simulink model "ANCfb"  (R2023b)
settings: Solver=ode3  StartTime=0.0  StopTime=10  RelTol=1e-3  EnableMultiTasking=on
libraries: matrix_library x52, dspadpt3 x31, raspberrypiAVlib x3
(part 1 of 2)
settings Model: FPTRunName=Active  ExtModeTrigDuration=2  Creator=aaron  LastModifiedBy=aaron
settings SolverCC: AlgebraicLoopSolver=TrustRegion  PositivePriorityOrder=on
settings DataIOCC: LimitDataPoints=on  SaveFormat=Array
settings OptimizationCC: ExpressionDepthLimit=2147483647  LifeSpan=Inf  MaxStackSize=64
settings DebuggingCC: UnderspecifiedInitializationDetection=Classic  MergeDetectMultiDrivingBlocksExec=none  FcnCallInpInsideContextMsg=warning  UnconnectedInputMsg=warning  UnconnectedOutputMsg=warning  UnconnectedLineMsg=warning  AllowSymbolicDim=off  StateNameClashWarn=warning  SubsystemReferenceDiagnosticForUnitTest=warning  SFUnexpectedBacktrackingDiag=warning  SFNoUnconditionalDefaultTransitionDiag=warning  SFExecutionAtInitializationDiag=none  ArithmeticOperatorsInVariantConditions=warning
settings HardwareCC: ProdBitPerPointer=32  ProdBitPerSizeT=32  ProdBitPerPtrDiffT=32  ProdLargestAtomicInteger=Long  ProdLargestAtomicFloat=Double  ProdWordSize=32  ProdHWDeviceType=ARM Compatible->ARM Cortex  UseEmbeddedCoderFeatures=off  UseSimulinkCoderFeatures=off
settings ModelReferenceCC: EnableRefExpFcnMdlSchedulingChecks=on  PropagateSignalLabelsOutOfModel=off
settings SFSimCC: SimUseLocalCustomCode=off  CustomCodeUndefinedFunction=UseInterfaceOnly
settings RTWCC: Description=Embedded Coder  SystemTargetFile=ert.tlc  HardwareBoard=Raspberry Pi  TemplateMakefile=ert_default_tmf  GenerateReport=on  RTWVerbose=off  RTWUseLocalCustomCode=off  Toolchain=GNU GCC Embedded Linux  BuildConfiguration=Faster Runs  LaunchReport=on
settings CodeAppCC: ForceParamTrailComments=on  OperatorAnnotations=on  StateflowObjectComments=on  MATLABSourceComments=on
settings ERTTargetCC: MultiwordLength=2048  ERTCustomFileBanners=off  SupportContinuousTime=on  SupportNonInlinedSFcns=on  RemoveResetFunc=off  SupportVariableSizeSignals=on  ModelStepFunctionPrototypeControlCompliant=off
settings ConfigComp: CovMetricSettings=dw  CovSaveCumulativeToWorkspaceVar=on  CovSaveSingleToWorkspaceVar=on  CovExternalEMLEnable=off  CovSFcnEnable=off

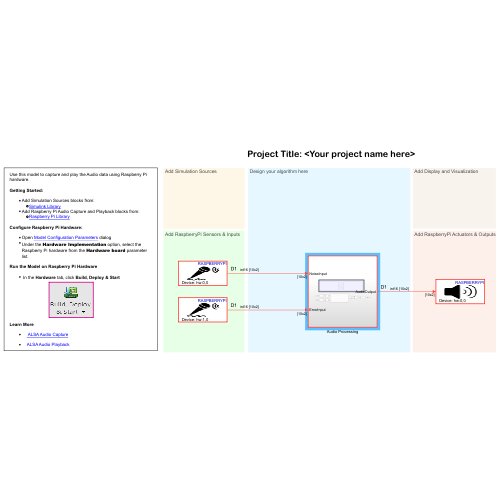
[thumbnail: Simulink's stored preview of the top-level diagram]
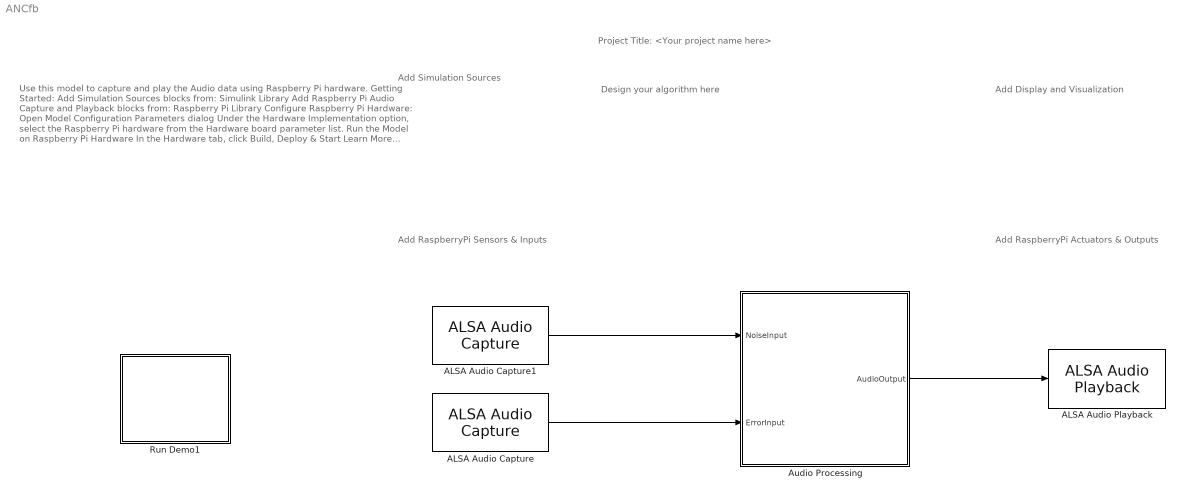
== system ANCfb ==
  note: Use this model to capture and play the Audio data using Raspberry Pi hardware.
      |
      | Getting Started:
      |
      | Add Simulation Sources blocks from:
      | Simulink Library
      | Add Raspberry Pi Audio Capture and Playback blocks from:
      | Raspberry Pi Library
      |
      | Configure Raspberry Pi Hardware:
      |
      | Open Model Configuration Parameters dialog
      | Under the Hardware Implementation option, select the Raspberry Pi hardware from the Hardware board parameter list.
      |
      | Run the Model on Raspberry Pi Hardware
      |
      | In the Hardware tab, click Build, Deploy & Start
      |
      | Learn More
      | ALSA Audio Capture
      | ALSA Audio Playback
  note: Add Simulation Sources
  note: Add Display and Visualization
  note: Design your algorithm here
  note: Add RaspberryPi Actuators & Outputs
  note: Project Title: <Your project name here>
  note: Add RaspberryPi Sensors & Inputs
  ALSA Audio Capture : raspberrypiAVlib/ALSA Audio Capture  deviceStr='hw:1,0'  DataBitDepth=16-bit integer  numberOfChannels=2  sampleRateEnum=44100  frameSize=10  QueueDuration=0.5  blockPlatform=Raspberry Pi
  ALSA Audio Capture1 : raspberrypiAVlib/ALSA Audio Capture  deviceStr='hw:0,0'  DataBitDepth=16-bit integer  numberOfChannels=2  sampleRateEnum=44100  frameSize=10  QueueDuration=0.5  blockPlatform=Raspberry Pi
  ALSA Audio Playback : raspberrypiAVlib/ALSA Audio Playback  deviceStr='hw:0,0'  sampleRateEnum=44100  queueDuration=0.5  blockPlatform=Raspberry Pi
  Audio Processing : Subsystem
  Run Demo1 : Subsystem  Description=Controls host-side RTDX processing.
      mask Display: pic=imread('raspberrypiBuildDeployAndStart.png');image(pic);
  wires:
  Audio Processing/1(AudioOutput) -> ALSA Audio Playback/1
  ALSA Audio Capture1/1 -> Audio Processing/1(NoiseInput)
  ALSA Audio Capture/1 -> Audio Processing/2(ErrorInput)

== system ANCfb/Audio Processing ==
  note: Unused Blocks
  NoiseInput : Inport
  ErrorInput : Inport  Port=2
  Data Type Conversion : DataTypeConversion  OutDataTypeStr=double  SaturateOnIntegerOverflow=off  RndMeth=Floor
  Data Type Conversion1 : DataTypeConversion  OutDataTypeStr=int16  SaturateOnIntegerOverflow=off  RndMeth=Floor  LockScale=on
  Data Type Conversion2 : DataTypeConversion  OutDataTypeStr=double  SaturateOnIntegerOverflow=off  RndMeth=Floor
  Frame Breakdown : Subsystem  TreatAsAtomicUnit=on
  Matrix Concatenate : Concatenate  Mode=Multidimensional array  ConcatenateDimension=2
  NoError : Subsystem  Commented=on  TreatAsAtomicUnit=on
  "Right Channel, exec" : Subsystem  Commented=on  TreatAsAtomicUnit=on
  Submatrix : matrix_library/Submatrix  RowSpan=All rows  RowStartMode=First  RowStartIndex=1  RowEndMode=Last  RowEndIndex=1  ColSpan=One column  ColStartMode=First  ColStartIndex=1  ColEndMode=Last  ColEndIndex=1
  Submatrix2 : matrix_library/Submatrix  RowSpan=All rows  RowStartMode=First  RowStartIndex=1  RowEndMode=Last  RowEndIndex=1  ColSpan=One column  ColStartMode=First  ColStartIndex=1  ColEndMode=Last  ColEndIndex=1
  AudioOutput : Outport
  wires:
  Data Type Conversion/1 -> Submatrix/1
  Submatrix/1 -> Frame Breakdown/1(Noise input (ref. mic.))
  NoiseInput/1 -> Data Type Conversion/1
  Data Type Conversion1/1 -> AudioOutput/1
  Frame Breakdown/1(Anti-noise output) -> Matrix Concatenate/2, Matrix Concatenate/1
  ErrorInput/1 -> Data Type Conversion2/1
  Data Type Conversion2/1 -> Submatrix2/1
  Submatrix2/1 -> Frame Breakdown/2(Error mic)
  Matrix Concatenate/1 -> Data Type Conversion1/1

== system ANCfb/Run Demo1 ==

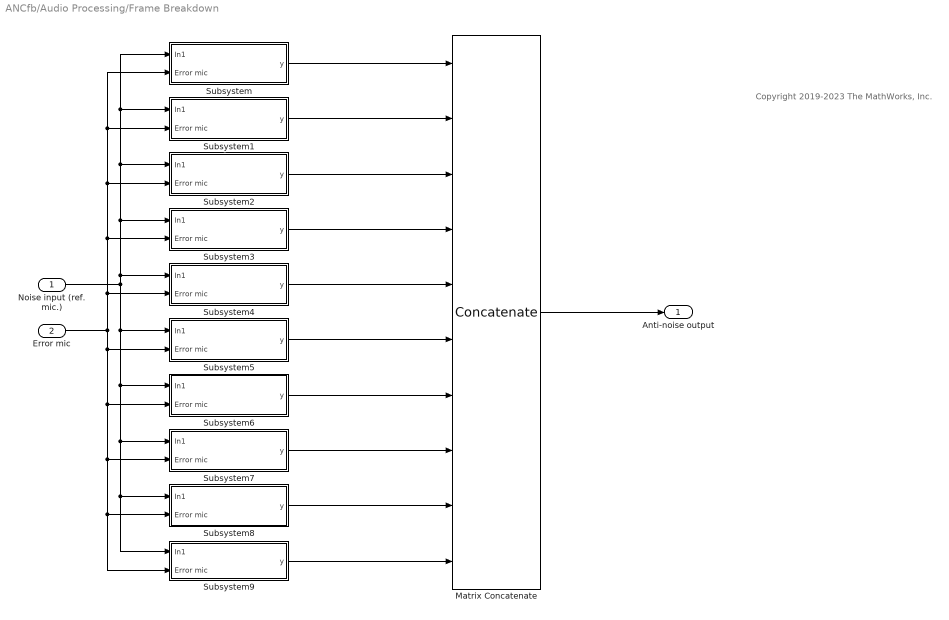
== system ANCfb/Audio Processing/Frame Breakdown ==
  note: Copyright 2019-2023 The MathWorks, Inc.
  Noise input (ref. mic.) : Inport
  Error mic : Inport  Port=2
  Matrix Concatenate : Concatenate  NumInputs=10  Mode=Multidimensional array
  Subsystem : Subsystem
  Subsystem1 : Subsystem
  Subsystem2 : Subsystem
  Subsystem3 : Subsystem
  Subsystem4 : Subsystem
  Subsystem5 : Subsystem
  Subsystem6 : Subsystem
  Subsystem7 : Subsystem
  Subsystem8 : Subsystem
  Subsystem9 : Subsystem
  Anti-noise output : Outport
  wires:
  Noise input (ref. mic.)/1 -> Subsystem4/1(In1), Subsystem3/1(In1), Subsystem2/1(In1), Subsystem1/1(In1), Subsystem/1(In1), Subsystem9/1(In1), Subsystem8/1(In1), Subsystem7/1(In1), Subsystem6/1(In1), Subsystem5/1(In1)
  Matrix Concatenate/1 -> Anti-noise output/1
  Subsystem/1(y) -> Matrix Concatenate/1
  Subsystem1/1(y) -> Matrix Concatenate/2
  Subsystem2/1(y) -> Matrix Concatenate/3
  Subsystem3/1(y) -> Matrix Concatenate/4
  Subsystem4/1(y) -> Matrix Concatenate/5
  Subsystem5/1(y) -> Matrix Concatenate/6
  Subsystem6/1(y) -> Matrix Concatenate/7
  Subsystem7/1(y) -> Matrix Concatenate/8
  Subsystem8/1(y) -> Matrix Concatenate/9
  Subsystem9/1(y) -> Matrix Concatenate/10
  Error mic/1 -> Subsystem9/2(Error mic), Subsystem8/2(Error mic), Subsystem7/2(Error mic), Subsystem6/2(Error mic), Subsystem5/2(Error mic), Subsystem4/2(Error mic), Subsystem1/2(Error mic), Subsystem/2(Error mic), Subsystem2/2(Error mic), Subsystem3/2(Error mic)

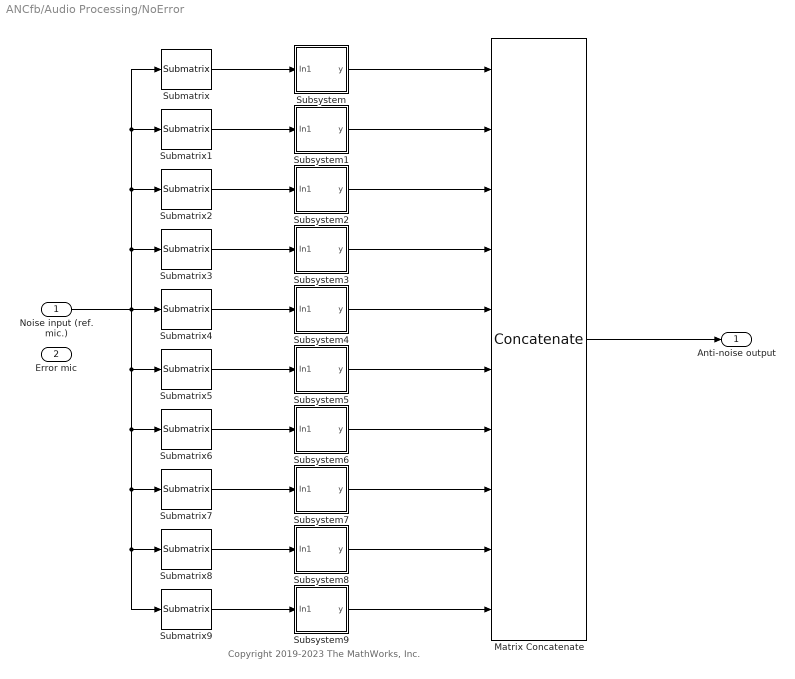
== system ANCfb/Audio Processing/NoError ==
  note: Copyright 2019-2023 The MathWorks, Inc.
  Noise input (ref. mic.) : Inport
  Error mic : Inport  Port=2
  Matrix Concatenate : Concatenate  NumInputs=10  Mode=Multidimensional array
  Submatrix : matrix_library/Submatrix  RowSpan=One row  RowStartMode=Index  RowStartIndex=1  RowEndMode=Last  RowEndIndex=1  ColSpan=One column  ColStartMode=First  ColStartIndex=1  ColEndMode=Last  ColEndIndex=1
  Submatrix1 : matrix_library/Submatrix  RowSpan=One row  RowStartMode=Index  RowStartIndex=2  RowEndMode=Last  RowEndIndex=1  ColSpan=One column  ColStartMode=First  ColStartIndex=1  ColEndMode=Last  ColEndIndex=1
  Submatrix2 : matrix_library/Submatrix  RowSpan=One row  RowStartMode=Index  RowStartIndex=3  RowEndMode=Last  RowEndIndex=1  ColSpan=One column  ColStartMode=First  ColStartIndex=1  ColEndMode=Last  ColEndIndex=1
  Submatrix3 : matrix_library/Submatrix  RowSpan=One row  RowStartMode=Index  RowStartIndex=4  RowEndMode=Last  RowEndIndex=1  ColSpan=One column  ColStartMode=First  ColStartIndex=1  ColEndMode=Last  ColEndIndex=1
  Submatrix4 : matrix_library/Submatrix  RowSpan=One row  RowStartMode=Index  RowStartIndex=5  RowEndMode=Last  RowEndIndex=1  ColSpan=One column  ColStartMode=First  ColStartIndex=1  ColEndMode=Last  ColEndIndex=1
  Submatrix5 : matrix_library/Submatrix  RowSpan=One row  RowStartMode=Index  RowStartIndex=6  RowEndMode=Last  RowEndIndex=1  ColSpan=One column  ColStartMode=First  ColStartIndex=1  ColEndMode=Last  ColEndIndex=1
  Submatrix6 : matrix_library/Submatrix  RowSpan=One row  RowStartMode=Index  RowStartIndex=7  RowEndMode=Last  RowEndIndex=1  ColSpan=One column  ColStartMode=First  ColStartIndex=1  ColEndMode=Last  ColEndIndex=1
  Submatrix7 : matrix_library/Submatrix  RowSpan=One row  RowStartMode=Index  RowStartIndex=8  RowEndMode=Last  RowEndIndex=1  ColSpan=One column  ColStartMode=First  ColStartIndex=1  ColEndMode=Last  ColEndIndex=1
  Submatrix8 : matrix_library/Submatrix  RowSpan=One row  RowStartMode=Index  RowStartIndex=9  RowEndMode=Last  RowEndIndex=1  ColSpan=One column  ColStartMode=First  ColStartIndex=1  ColEndMode=Last  ColEndIndex=1
  Submatrix9 : matrix_library/Submatrix  RowSpan=One row  RowStartMode=Index  RowStartIndex=10  RowEndMode=Last  RowEndIndex=1  ColSpan=One column  ColStartMode=First  ColStartIndex=1  ColEndMode=Last  ColEndIndex=1
  Subsystem : Subsystem
  Subsystem1 : Subsystem
  Subsystem2 : Subsystem
  Subsystem3 : Subsystem
  Subsystem4 : Subsystem
  Subsystem5 : Subsystem
  Subsystem6 : Subsystem
  Subsystem7 : Subsystem
  Subsystem8 : Subsystem
  Subsystem9 : Subsystem
  Anti-noise output : Outport
  wires:
  Submatrix1/1 -> Subsystem1/1(In1)
  Submatrix2/1 -> Subsystem2/1(In1)
  Submatrix3/1 -> Subsystem3/1(In1)
  Submatrix4/1 -> Subsystem4/1(In1)
  Submatrix5/1 -> Subsystem5/1(In1)
  Submatrix6/1 -> Subsystem6/1(In1)
  Submatrix7/1 -> Subsystem7/1(In1)
  Submatrix8/1 -> Subsystem8/1(In1)
  Submatrix9/1 -> Subsystem9/1(In1)
  Noise input (ref. mic.)/1 -> Submatrix9/1, Submatrix8/1, Submatrix7/1, Submatrix6/1, Submatrix5/1, Submatrix/1, Submatrix1/1, Submatrix2/1, Submatrix3/1, Submatrix4/1
  Subsystem1/1(y) -> Matrix Concatenate/2
  Subsystem2/1(y) -> Matrix Concatenate/3
  Subsystem3/1(y) -> Matrix Concatenate/4
  Subsystem4/1(y) -> Matrix Concatenate/5
  Subsystem5/1(y) -> Matrix Concatenate/6
  Matrix Concatenate/1 -> Anti-noise output/1
  Subsystem6/1(y) -> Matrix Concatenate/7
  Subsystem7/1(y) -> Matrix Concatenate/8
  Subsystem8/1(y) -> Matrix Concatenate/9
  Subsystem9/1(y) -> Matrix Concatenate/10
  Submatrix/1 -> Subsystem/1(In1)
  Subsystem/1(y) -> Matrix Concatenate/1

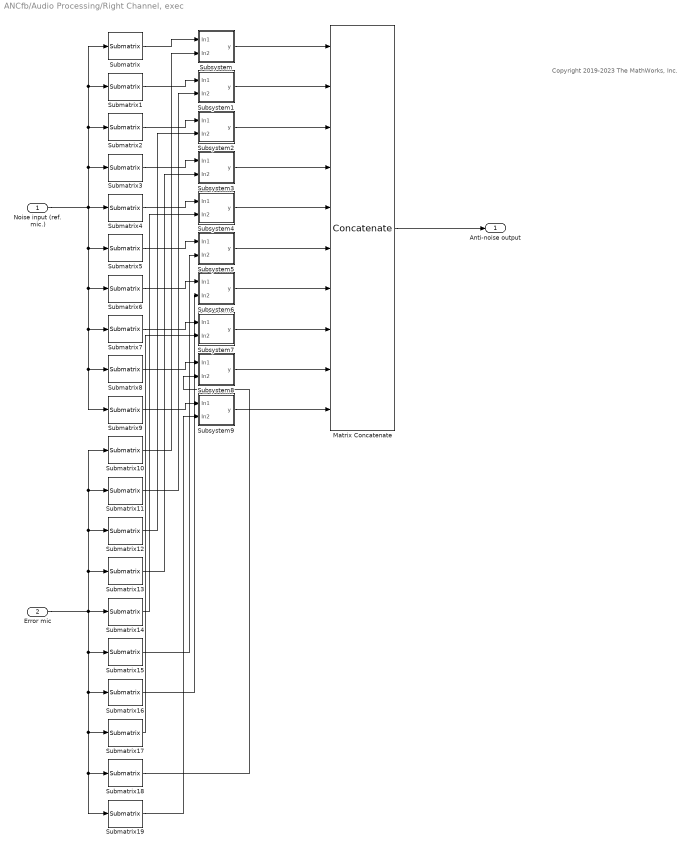
== system ANCfb/Audio Processing/Right Channel, exec ==
  note: Copyright 2019-2023 The MathWorks, Inc.
  Noise input (ref. mic.) : Inport
  Error mic : Inport  Port=2
  Matrix Concatenate : Concatenate  NumInputs=10  Mode=Multidimensional array
  Submatrix : matrix_library/Submatrix  RowSpan=One row  RowStartMode=Index  RowStartIndex=1  RowEndMode=Last  RowEndIndex=1  ColSpan=One column  ColStartMode=First  ColStartIndex=1  ColEndMode=Last  ColEndIndex=1
  Submatrix1 : matrix_library/Submatrix  RowSpan=One row  RowStartMode=Index  RowStartIndex=2  RowEndMode=Last  RowEndIndex=1  ColSpan=One column  ColStartMode=First  ColStartIndex=1  ColEndMode=Last  ColEndIndex=1
  Submatrix10 : matrix_library/Submatrix  RowSpan=One row  RowStartMode=Index  RowStartIndex=1  RowEndMode=Last  RowEndIndex=1  ColSpan=One column  ColStartMode=First  ColStartIndex=1  ColEndMode=Last  ColEndIndex=1
  Submatrix11 : matrix_library/Submatrix  RowSpan=One row  RowStartMode=Index  RowStartIndex=2  RowEndMode=Last  RowEndIndex=1  ColSpan=One column  ColStartMode=First  ColStartIndex=1  ColEndMode=Last  ColEndIndex=1
  Submatrix12 : matrix_library/Submatrix  RowSpan=One row  RowStartMode=Index  RowStartIndex=3  RowEndMode=Last  RowEndIndex=1  ColSpan=One column  ColStartMode=First  ColStartIndex=1  ColEndMode=Last  ColEndIndex=1
  Submatrix13 : matrix_library/Submatrix  RowSpan=One row  RowStartMode=Index  RowStartIndex=4  RowEndMode=Last  RowEndIndex=1  ColSpan=One column  ColStartMode=First  ColStartIndex=1  ColEndMode=Last  ColEndIndex=1
  Submatrix14 : matrix_library/Submatrix  RowSpan=One row  RowStartMode=Index  RowStartIndex=5  RowEndMode=Last  RowEndIndex=1  ColSpan=One column  ColStartMode=First  ColStartIndex=1  ColEndMode=Last  ColEndIndex=1
  Submatrix15 : matrix_library/Submatrix  RowSpan=One row  RowStartMode=Index  RowStartIndex=6  RowEndMode=Last  RowEndIndex=1  ColSpan=One column  ColStartMode=First  ColStartIndex=1  ColEndMode=Last  ColEndIndex=1
  Submatrix16 : matrix_library/Submatrix  RowSpan=One row  RowStartMode=Index  RowStartIndex=7  RowEndMode=Last  RowEndIndex=1  ColSpan=One column  ColStartMode=First  ColStartIndex=1  ColEndMode=Last  ColEndIndex=1
  Submatrix17 : matrix_library/Submatrix  RowSpan=One row  RowStartMode=Index  RowStartIndex=8  RowEndMode=Last  RowEndIndex=1  ColSpan=One column  ColStartMode=First  ColStartIndex=1  ColEndMode=Last  ColEndIndex=1
  Submatrix18 : matrix_library/Submatrix  RowSpan=One row  RowStartMode=Index  RowStartIndex=9  RowEndMode=Last  RowEndIndex=1  ColSpan=One column  ColStartMode=First  ColStartIndex=1  ColEndMode=Last  ColEndIndex=1
  Submatrix19 : matrix_library/Submatrix  RowSpan=One row  RowStartMode=Index  RowStartIndex=10  RowEndMode=Last  RowEndIndex=1  ColSpan=One column  ColStartMode=First  ColStartIndex=1  ColEndMode=Last  ColEndIndex=1
  Submatrix2 : matrix_library/Submatrix  RowSpan=One row  RowStartMode=Index  RowStartIndex=3  RowEndMode=Last  RowEndIndex=1  ColSpan=One column  ColStartMode=First  ColStartIndex=1  ColEndMode=Last  ColEndIndex=1
  Submatrix3 : matrix_library/Submatrix  RowSpan=One row  RowStartMode=Index  RowStartIndex=4  RowEndMode=Last  RowEndIndex=1  ColSpan=One column  ColStartMode=First  ColStartIndex=1  ColEndMode=Last  ColEndIndex=1
  Submatrix4 : matrix_library/Submatrix  RowSpan=One row  RowStartMode=Index  RowStartIndex=5  RowEndMode=Last  RowEndIndex=1  ColSpan=One column  ColStartMode=First  ColStartIndex=1  ColEndMode=Last  ColEndIndex=1
  Submatrix5 : matrix_library/Submatrix  RowSpan=One row  RowStartMode=Index  RowStartIndex=6  RowEndMode=Last  RowEndIndex=1  ColSpan=One column  ColStartMode=First  ColStartIndex=1  ColEndMode=Last  ColEndIndex=1
  Submatrix6 : matrix_library/Submatrix  RowSpan=One row  RowStartMode=Index  RowStartIndex=7  RowEndMode=Last  RowEndIndex=1  ColSpan=One column  ColStartMode=First  ColStartIndex=1  ColEndMode=Last  ColEndIndex=1
  Submatrix7 : matrix_library/Submatrix  RowSpan=One row  RowStartMode=Index  RowStartIndex=8  RowEndMode=Last  RowEndIndex=1  ColSpan=One column  ColStartMode=First  ColStartIndex=1  ColEndMode=Last  ColEndIndex=1
  Submatrix8 : matrix_library/Submatrix  RowSpan=One row  RowStartMode=Index  RowStartIndex=9  RowEndMode=Last  RowEndIndex=1  ColSpan=One column  ColStartMode=First  ColStartIndex=1  ColEndMode=Last  ColEndIndex=1
  Submatrix9 : matrix_library/Submatrix  RowSpan=One row  RowStartMode=Index  RowStartIndex=10  RowEndMode=Last  RowEndIndex=1  ColSpan=One column  ColStartMode=First  ColStartIndex=1  ColEndMode=Last  ColEndIndex=1
  Subsystem : Subsystem
  Subsystem1 : Subsystem
  Subsystem2 : Subsystem
  Subsystem3 : Subsystem
  Subsystem4 : Subsystem
  Subsystem5 : Subsystem
  Subsystem6 : Subsystem
  Subsystem7 : Subsystem
  Subsystem8 : Subsystem
  Subsystem9 : Subsystem
  Anti-noise output : Outport
  wires:
  Submatrix1/1 -> Subsystem1/1(In1)
  Submatrix2/1 -> Subsystem2/1(In1)
  Submatrix3/1 -> Subsystem3/1(In1)
  Submatrix4/1 -> Subsystem4/1(In1)
  Submatrix5/1 -> Subsystem5/1(In1)
  Submatrix6/1 -> Subsystem6/1(In1)
  Submatrix7/1 -> Subsystem7/1(In1)
  Submatrix8/1 -> Subsystem8/1(In1)
  Submatrix9/1 -> Subsystem9/1(In1)
  Noise input (ref. mic.)/1 -> Submatrix9/1, Submatrix8/1, Submatrix7/1, Submatrix6/1, Submatrix5/1, Submatrix/1, Submatrix1/1, Submatrix2/1, Submatrix3/1, Submatrix4/1
  Subsystem1/1(y) -> Matrix Concatenate/2
  Subsystem2/1(y) -> Matrix Concatenate/3
  Subsystem3/1(y) -> Matrix Concatenate/4
  Subsystem4/1(y) -> Matrix Concatenate/5
  Subsystem5/1(y) -> Matrix Concatenate/6
  Matrix Concatenate/1 -> Anti-noise output/1
  Subsystem6/1(y) -> Matrix Concatenate/7
  Subsystem7/1(y) -> Matrix Concatenate/8
  Subsystem8/1(y) -> Matrix Concatenate/9
  Subsystem9/1(y) -> Matrix Concatenate/10
  Submatrix/1 -> Subsystem/1(In1)
  Subsystem/1(y) -> Matrix Concatenate/1
  Error mic/1 -> Submatrix19/1, Submatrix18/1, Submatrix17/1, Submatrix16/1, Submatrix15/1, Submatrix10/1, Submatrix11/1, Submatrix12/1, Submatrix13/1, Submatrix14/1
  Submatrix10/1 -> Subsystem/2(In2)
  Submatrix11/1 -> Subsystem1/2(In2)
  Submatrix12/1 -> Subsystem2/2(In2)
  Submatrix13/1 -> Subsystem3/2(In2)
  Submatrix14/1 -> Subsystem4/2(In2)
  Submatrix15/1 -> Subsystem5/2(In2)
  Submatrix16/1 -> Subsystem6/2(In2)
  Submatrix17/1 -> Subsystem7/2(In2)
  Submatrix18/1 -> Subsystem8/2(In2)
  Submatrix19/1 -> Subsystem9/2(In2)

== system ANCfb/Audio Processing/Frame Breakdown/Subsystem ==
  In1 : Inport
  Error mic : Inport  Port=2
  Submatrix : matrix_library/Submatrix  RowSpan=One row  RowStartMode=Index  RowStartIndex=1  RowEndMode=Last  RowEndIndex=1  ColSpan=One column  ColStartMode=First  ColStartIndex=1  ColEndMode=Last  ColEndIndex=1
  Submatrix10 : matrix_library/Submatrix  RowSpan=One row  RowStartMode=Index  RowStartIndex=1  RowEndMode=Last  RowEndIndex=1  ColSpan=One column  ColStartMode=First  ColStartIndex=1  ColEndMode=Last  ColEndIndex=1
  Subsystem : Subsystem
  y : Outport
  wires:
  Error mic/1 -> Submatrix10/1
  Submatrix/1 -> Subsystem/1(In1)
  Submatrix10/1 -> Subsystem/2(In2)
  In1/1 -> Submatrix/1
  Subsystem/1(y) -> y/1

== system ANCfb/Audio Processing/Frame Breakdown/Subsystem1 ==
  In1 : Inport
  Error mic : Inport  Port=2
  Submatrix1 : matrix_library/Submatrix  RowSpan=One row  RowStartMode=Index  RowStartIndex=2  RowEndMode=Last  RowEndIndex=1  ColSpan=One column  ColStartMode=First  ColStartIndex=1  ColEndMode=Last  ColEndIndex=1
  Submatrix11 : matrix_library/Submatrix  RowSpan=One row  RowStartMode=Index  RowStartIndex=2  RowEndMode=Last  RowEndIndex=1  ColSpan=One column  ColStartMode=First  ColStartIndex=1  ColEndMode=Last  ColEndIndex=1
  Subsystem1 : Subsystem
  y : Outport
  wires:
  Submatrix1/1 -> Subsystem1/1(In1)
  Error mic/1 -> Submatrix11/1
  In1/1 -> Submatrix1/1
  Submatrix11/1 -> Subsystem1/2(In2)
  Subsystem1/1(y) -> y/1

== system ANCfb/Audio Processing/Frame Breakdown/Subsystem2 ==
  In1 : Inport
  Error mic : Inport  Port=2
  Submatrix12 : matrix_library/Submatrix  RowSpan=One row  RowStartMode=Index  RowStartIndex=3  RowEndMode=Last  RowEndIndex=1  ColSpan=One column  ColStartMode=First  ColStartIndex=1  ColEndMode=Last  ColEndIndex=1
  Submatrix2 : matrix_library/Submatrix  RowSpan=One row  RowStartMode=Index  RowStartIndex=3  RowEndMode=Last  RowEndIndex=1  ColSpan=One column  ColStartMode=First  ColStartIndex=1  ColEndMode=Last  ColEndIndex=1
  Subsystem2 : Subsystem
  y : Outport
  wires:
  Submatrix12/1 -> Subsystem2/2(In2)
  Error mic/1 -> Submatrix12/1
  Submatrix2/1 -> Subsystem2/1(In1)
  Subsystem2/1(y) -> y/1
  In1/1 -> Submatrix2/1

== system ANCfb/Audio Processing/Frame Breakdown/Subsystem3 ==
  In1 : Inport
  Error mic : Inport  Port=2
  Submatrix13 : matrix_library/Submatrix  RowSpan=One row  RowStartMode=Index  RowStartIndex=4  RowEndMode=Last  RowEndIndex=1  ColSpan=One column  ColStartMode=First  ColStartIndex=1  ColEndMode=Last  ColEndIndex=1
  Submatrix3 : matrix_library/Submatrix  RowSpan=One row  RowStartMode=Index  RowStartIndex=4  RowEndMode=Last  RowEndIndex=1  ColSpan=One column  ColStartMode=First  ColStartIndex=1  ColEndMode=Last  ColEndIndex=1
  Subsystem3 : Subsystem
  y : Outport
  wires:
  Subsystem3/1(y) -> y/1
  Submatrix13/1 -> Subsystem3/2(In2)
  In1/1 -> Submatrix3/1
  Submatrix3/1 -> Subsystem3/1(In1)
  Error mic/1 -> Submatrix13/1

== system ANCfb/Audio Processing/Frame Breakdown/Subsystem4 ==
  In1 : Inport
  Error mic : Inport  Port=2
  Submatrix14 : matrix_library/Submatrix  RowSpan=One row  RowStartMode=Index  RowStartIndex=5  RowEndMode=Last  RowEndIndex=1  ColSpan=One column  ColStartMode=First  ColStartIndex=1  ColEndMode=Last  ColEndIndex=1
  Submatrix4 : matrix_library/Submatrix  RowSpan=One row  RowStartMode=Index  RowStartIndex=5  RowEndMode=Last  RowEndIndex=1  ColSpan=One column  ColStartMode=First  ColStartIndex=1  ColEndMode=Last  ColEndIndex=1
  Subsystem4 : Subsystem
  y : Outport
  wires:
  Subsystem4/1(y) -> y/1
  Error mic/1 -> Submatrix14/1
  Submatrix14/1 -> Subsystem4/2(In2)
  Submatrix4/1 -> Subsystem4/1(In1)
  In1/1 -> Submatrix4/1

== system ANCfb/Audio Processing/Frame Breakdown/Subsystem5 ==
  In1 : Inport
  Error mic : Inport  Port=2
  Submatrix15 : matrix_library/Submatrix  RowSpan=One row  RowStartMode=Index  RowStartIndex=6  RowEndMode=Last  RowEndIndex=1  ColSpan=One column  ColStartMode=First  ColStartIndex=1  ColEndMode=Last  ColEndIndex=1
  Submatrix5 : matrix_library/Submatrix  RowSpan=One row  RowStartMode=Index  RowStartIndex=6  RowEndMode=Last  RowEndIndex=1  ColSpan=One column  ColStartMode=First  ColStartIndex=1  ColEndMode=Last  ColEndIndex=1
  Subsystem5 : Subsystem
  y : Outport
  wires:
  Submatrix15/1 -> Subsystem5/2(In2)
  Error mic/1 -> Submatrix15/1
  Submatrix5/1 -> Subsystem5/1(In1)
  In1/1 -> Submatrix5/1
  Subsystem5/1(y) -> y/1

== system ANCfb/Audio Processing/Frame Breakdown/Subsystem6 ==
  In1 : Inport
  Error mic : Inport  Port=2
  Submatrix16 : matrix_library/Submatrix  RowSpan=One row  RowStartMode=Index  RowStartIndex=7  RowEndMode=Last  RowEndIndex=1  ColSpan=One column  ColStartMode=First  ColStartIndex=1  ColEndMode=Last  ColEndIndex=1
  Submatrix6 : matrix_library/Submatrix  RowSpan=One row  RowStartMode=Index  RowStartIndex=7  RowEndMode=Last  RowEndIndex=1  ColSpan=One column  ColStartMode=First  ColStartIndex=1  ColEndMode=Last  ColEndIndex=1
  Subsystem6 : Subsystem
  y : Outport
  wires:
  Submatrix6/1 -> Subsystem6/1(In1)
  Submatrix16/1 -> Subsystem6/2(In2)
  Subsystem6/1(y) -> y/1
  In1/1 -> Submatrix6/1
  Error mic/1 -> Submatrix16/1

== system ANCfb/Audio Processing/Frame Breakdown/Subsystem7 ==
  In1 : Inport
  Error mic : Inport  Port=2
  Submatrix17 : matrix_library/Submatrix  RowSpan=One row  RowStartMode=Index  RowStartIndex=8  RowEndMode=Last  RowEndIndex=1  ColSpan=One column  ColStartMode=First  ColStartIndex=1  ColEndMode=Last  ColEndIndex=1
  Submatrix7 : matrix_library/Submatrix  RowSpan=One row  RowStartMode=Index  RowStartIndex=8  RowEndMode=Last  RowEndIndex=1  ColSpan=One column  ColStartMode=First  ColStartIndex=1  ColEndMode=Last  ColEndIndex=1
  Subsystem7 : Subsystem
  y : Outport
  wires:
  Submatrix7/1 -> Subsystem7/1(In1)
  Submatrix17/1 -> Subsystem7/2(In2)
  In1/1 -> Submatrix7/1
  Subsystem7/1(y) -> y/1
  Error mic/1 -> Submatrix17/1

== system ANCfb/Audio Processing/Frame Breakdown/Subsystem8 ==
  In1 : Inport
  Error mic : Inport  Port=2
  Submatrix18 : matrix_library/Submatrix  RowSpan=One row  RowStartMode=Index  RowStartIndex=9  RowEndMode=Last  RowEndIndex=1  ColSpan=One column  ColStartMode=First  ColStartIndex=1  ColEndMode=Last  ColEndIndex=1
  Submatrix8 : matrix_library/Submatrix  RowSpan=One row  RowStartMode=Index  RowStartIndex=9  RowEndMode=Last  RowEndIndex=1  ColSpan=One column  ColStartMode=First  ColStartIndex=1  ColEndMode=Last  ColEndIndex=1
  Subsystem8 : Subsystem
  y : Outport
  wires:
  Subsystem8/1(y) -> y/1
  Submatrix18/1 -> Subsystem8/2(In2)
  In1/1 -> Submatrix8/1
  Submatrix8/1 -> Subsystem8/1(In1)
  Error mic/1 -> Submatrix18/1

== system ANCfb/Audio Processing/Frame Breakdown/Subsystem9 ==
  In1 : Inport
  Error mic : Inport  Port=2
  Submatrix19 : matrix_library/Submatrix  RowSpan=One row  RowStartMode=Index  RowStartIndex=10  RowEndMode=Last  RowEndIndex=1  ColSpan=One column  ColStartMode=First  ColStartIndex=1  ColEndMode=Last  ColEndIndex=1
  Submatrix9 : matrix_library/Submatrix  RowSpan=One row  RowStartMode=Index  RowStartIndex=10  RowEndMode=Last  RowEndIndex=1  ColSpan=One column  ColStartMode=First  ColStartIndex=1  ColEndMode=Last  ColEndIndex=1
  Subsystem9 : Subsystem
  y : Outport
  wires:
  Submatrix19/1 -> Subsystem9/2(In2)
  Submatrix9/1 -> Subsystem9/1(In1)
  Error mic/1 -> Submatrix19/1
  In1/1 -> Submatrix9/1
  Subsystem9/1(y) -> y/1

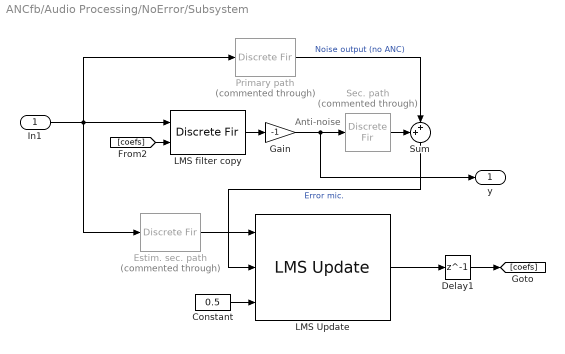
== system ANCfb/Audio Processing/NoError/Subsystem ==
  note: Anti-noise
  In1 : Inport
  Constant : Constant  Value=0.5
  Delay1 : Delay  DelayLength=1
  Estim. sec. path : DiscreteFir  Commented=through  Coefficients="[0.466  0.533  -0.257  -0.274  -0.231  -0.175]"
  Gain : Gain  Gain=-1
  LMS Update : dspadpt3/LMS Update  Method=Normalized LMS  Length=200  NumFilters=1  StepSizeSource=Input port  StepSize=0.1  LeakageFactor=1.0  InitialConditions=0  AdaptiveFilterMode=Tapped delay-line FIR filter  EnableAdaptInput=off  EnableResetInput=off  SimulateUsing=Interpreted execution
  LMS filter copy : DiscreteFir  CoefSource=Input port
      settings: InputPortMap=u0,u1
  Primary path : DiscreteFir  Commented=through  Coefficients=conv([0.5 0.5 -.3 -.3 -.2 -.2],[.1 -.1 .2 -.2 .3 -.3 .15 -.15])
  Sec. path : DiscreteFir  Commented=through  Coefficients=[0.5 0.5 -.3 -.3 -.2 -.2]
  Sum : Sum  Inputs=++|
  y : Outport
  wires:
  Primary path/1 -> Sum/2  "Noise output (no ANC)"
  Gain/1 -> y/1, Sec. path/1
  Constant/1 -> LMS Update/3
  LMS filter copy/1 -> Gain/1
  [coefs] -> LMS filter copy/2
  Sum/1 -> LMS Update/2  "Error mic."
  Delay1/1 -> [coefs]
  LMS Update/1 -> Delay1/1
  In1/1 -> Primary path/1, Estim. sec. path/1, LMS filter copy/1
  Estim. sec. path/1 -> LMS Update/1
  Sec. path/1 -> Sum/1

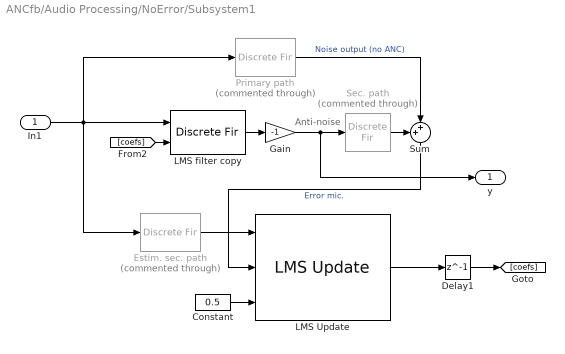
== system ANCfb/Audio Processing/NoError/Subsystem1 ==
  note: Anti-noise
  In1 : Inport
  Constant : Constant  Value=0.5
  Delay1 : Delay  DelayLength=1
  Estim. sec. path : DiscreteFir  Commented=through  Coefficients="[0.466  0.533  -0.257  -0.274  -0.231  -0.175]"
  Gain : Gain  Gain=-1
  LMS Update : dspadpt3/LMS Update  Method=Normalized LMS  Length=200  NumFilters=1  StepSizeSource=Input port  StepSize=0.1  LeakageFactor=1.0  InitialConditions=0  AdaptiveFilterMode=Tapped delay-line FIR filter  EnableAdaptInput=off  EnableResetInput=off  SimulateUsing=Interpreted execution
  LMS filter copy : DiscreteFir  CoefSource=Input port
      settings: InputPortMap=u0,u1
  Primary path : DiscreteFir  Commented=through  Coefficients=conv([0.5 0.5 -.3 -.3 -.2 -.2],[.1 -.1 .2 -.2 .3 -.3 .15 -.15])
  Sec. path : DiscreteFir  Commented=through  Coefficients=[0.5 0.5 -.3 -.3 -.2 -.2]
  Sum : Sum  Inputs=++|
  y : Outport
  wires:
  Primary path/1 -> Sum/2  "Noise output (no ANC)"
  Gain/1 -> y/1, Sec. path/1
  Constant/1 -> LMS Update/3
  LMS filter copy/1 -> Gain/1
  [coefs] -> LMS filter copy/2
  Sum/1 -> LMS Update/2  "Error mic."
  Delay1/1 -> [coefs]
  LMS Update/1 -> Delay1/1
  In1/1 -> Primary path/1, Estim. sec. path/1, LMS filter copy/1
  Estim. sec. path/1 -> LMS Update/1
  Sec. path/1 -> Sum/1

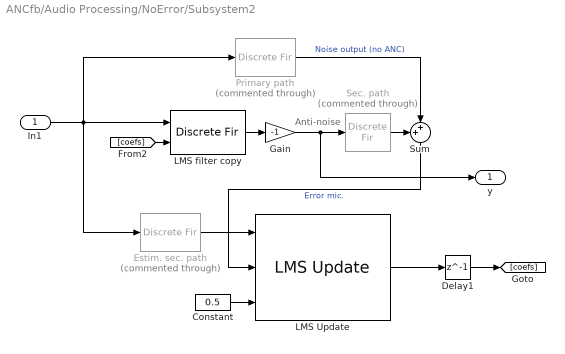
== system ANCfb/Audio Processing/NoError/Subsystem2 ==
  note: Anti-noise
  In1 : Inport
  Constant : Constant  Value=0.5
  Delay1 : Delay  DelayLength=1
  Estim. sec. path : DiscreteFir  Commented=through  Coefficients="[0.466  0.533  -0.257  -0.274  -0.231  -0.175]"
  Gain : Gain  Gain=-1
  LMS Update : dspadpt3/LMS Update  Method=Normalized LMS  Length=200  NumFilters=1  StepSizeSource=Input port  StepSize=0.1  LeakageFactor=1.0  InitialConditions=0  AdaptiveFilterMode=Tapped delay-line FIR filter  EnableAdaptInput=off  EnableResetInput=off  SimulateUsing=Interpreted execution
  LMS filter copy : DiscreteFir  CoefSource=Input port
      settings: InputPortMap=u0,u1
  Primary path : DiscreteFir  Commented=through  Coefficients=conv([0.5 0.5 -.3 -.3 -.2 -.2],[.1 -.1 .2 -.2 .3 -.3 .15 -.15])
  Sec. path : DiscreteFir  Commented=through  Coefficients=[0.5 0.5 -.3 -.3 -.2 -.2]
  Sum : Sum  Inputs=++|
  y : Outport
  wires:
  Primary path/1 -> Sum/2  "Noise output (no ANC)"
  Gain/1 -> y/1, Sec. path/1
  Constant/1 -> LMS Update/3
  LMS filter copy/1 -> Gain/1
  [coefs] -> LMS filter copy/2
  Sum/1 -> LMS Update/2  "Error mic."
  Delay1/1 -> [coefs]
  LMS Update/1 -> Delay1/1
  In1/1 -> Primary path/1, Estim. sec. path/1, LMS filter copy/1
  Estim. sec. path/1 -> LMS Update/1
  Sec. path/1 -> Sum/1

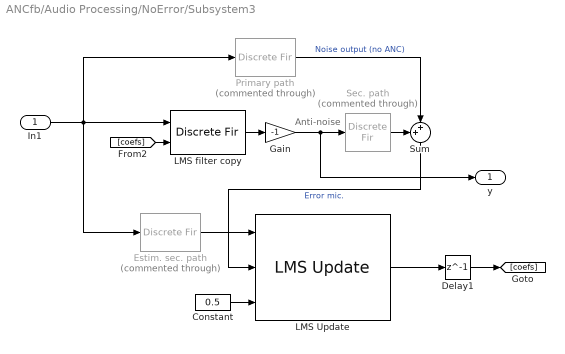
== system ANCfb/Audio Processing/NoError/Subsystem3 ==
  note: Anti-noise
  In1 : Inport
  Constant : Constant  Value=0.5
  Delay1 : Delay  DelayLength=1
  Estim. sec. path : DiscreteFir  Commented=through  Coefficients="[0.466  0.533  -0.257  -0.274  -0.231  -0.175]"
  Gain : Gain  Gain=-1
  LMS Update : dspadpt3/LMS Update  Method=Normalized LMS  Length=200  NumFilters=1  StepSizeSource=Input port  StepSize=0.1  LeakageFactor=1.0  InitialConditions=0  AdaptiveFilterMode=Tapped delay-line FIR filter  EnableAdaptInput=off  EnableResetInput=off  SimulateUsing=Interpreted execution
  LMS filter copy : DiscreteFir  CoefSource=Input port
      settings: InputPortMap=u0,u1
  Primary path : DiscreteFir  Commented=through  Coefficients=conv([0.5 0.5 -.3 -.3 -.2 -.2],[.1 -.1 .2 -.2 .3 -.3 .15 -.15])
  Sec. path : DiscreteFir  Commented=through  Coefficients=[0.5 0.5 -.3 -.3 -.2 -.2]
  Sum : Sum  Inputs=++|
  y : Outport
  wires:
  Primary path/1 -> Sum/2  "Noise output (no ANC)"
  Gain/1 -> y/1, Sec. path/1
  Constant/1 -> LMS Update/3
  LMS filter copy/1 -> Gain/1
  [coefs] -> LMS filter copy/2
  Sum/1 -> LMS Update/2  "Error mic."
  Delay1/1 -> [coefs]
  LMS Update/1 -> Delay1/1
  In1/1 -> Primary path/1, Estim. sec. path/1, LMS filter copy/1
  Estim. sec. path/1 -> LMS Update/1
  Sec. path/1 -> Sum/1

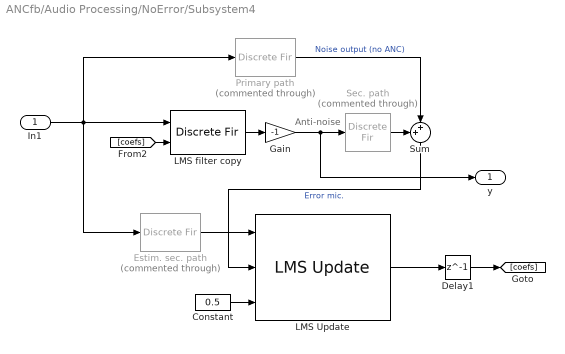
== system ANCfb/Audio Processing/NoError/Subsystem4 ==
  note: Anti-noise
  In1 : Inport
  Constant : Constant  Value=0.5
  Delay1 : Delay  DelayLength=1
  Estim. sec. path : DiscreteFir  Commented=through  Coefficients="[0.466  0.533  -0.257  -0.274  -0.231  -0.175]"
  Gain : Gain  Gain=-1
  LMS Update : dspadpt3/LMS Update  Method=Normalized LMS  Length=200  NumFilters=1  StepSizeSource=Input port  StepSize=0.1  LeakageFactor=1.0  InitialConditions=0  AdaptiveFilterMode=Tapped delay-line FIR filter  EnableAdaptInput=off  EnableResetInput=off  SimulateUsing=Interpreted execution
  LMS filter copy : DiscreteFir  CoefSource=Input port
      settings: InputPortMap=u0,u1
  Primary path : DiscreteFir  Commented=through  Coefficients=conv([0.5 0.5 -.3 -.3 -.2 -.2],[.1 -.1 .2 -.2 .3 -.3 .15 -.15])
  Sec. path : DiscreteFir  Commented=through  Coefficients=[0.5 0.5 -.3 -.3 -.2 -.2]
  Sum : Sum  Inputs=++|
  y : Outport
  wires:
  Primary path/1 -> Sum/2  "Noise output (no ANC)"
  Gain/1 -> y/1, Sec. path/1
  Constant/1 -> LMS Update/3
  LMS filter copy/1 -> Gain/1
  [coefs] -> LMS filter copy/2
  Sum/1 -> LMS Update/2  "Error mic."
  Delay1/1 -> [coefs]
  LMS Update/1 -> Delay1/1
  In1/1 -> Primary path/1, Estim. sec. path/1, LMS filter copy/1
  Estim. sec. path/1 -> LMS Update/1
  Sec. path/1 -> Sum/1

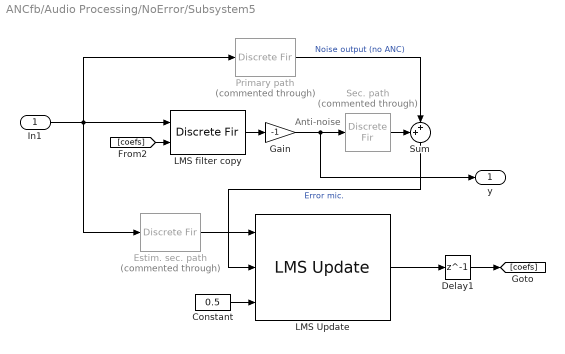
== system ANCfb/Audio Processing/NoError/Subsystem5 ==
  note: Anti-noise
  In1 : Inport
  Constant : Constant  Value=0.5
  Delay1 : Delay  DelayLength=1
  Estim. sec. path : DiscreteFir  Commented=through  Coefficients="[0.466  0.533  -0.257  -0.274  -0.231  -0.175]"
  Gain : Gain  Gain=-1
  LMS Update : dspadpt3/LMS Update  Method=Normalized LMS  Length=200  NumFilters=1  StepSizeSource=Input port  StepSize=0.1  LeakageFactor=1.0  InitialConditions=0  AdaptiveFilterMode=Tapped delay-line FIR filter  EnableAdaptInput=off  EnableResetInput=off  SimulateUsing=Interpreted execution
  LMS filter copy : DiscreteFir  CoefSource=Input port
      settings: InputPortMap=u0,u1
  Primary path : DiscreteFir  Commented=through  Coefficients=conv([0.5 0.5 -.3 -.3 -.2 -.2],[.1 -.1 .2 -.2 .3 -.3 .15 -.15])
  Sec. path : DiscreteFir  Commented=through  Coefficients=[0.5 0.5 -.3 -.3 -.2 -.2]
  Sum : Sum  Inputs=++|
  y : Outport
  wires:
  Primary path/1 -> Sum/2  "Noise output (no ANC)"
  Gain/1 -> y/1, Sec. path/1
  Constant/1 -> LMS Update/3
  LMS filter copy/1 -> Gain/1
  [coefs] -> LMS filter copy/2
  Sum/1 -> LMS Update/2  "Error mic."
  Delay1/1 -> [coefs]
  LMS Update/1 -> Delay1/1
  In1/1 -> Primary path/1, Estim. sec. path/1, LMS filter copy/1
  Estim. sec. path/1 -> LMS Update/1
  Sec. path/1 -> Sum/1

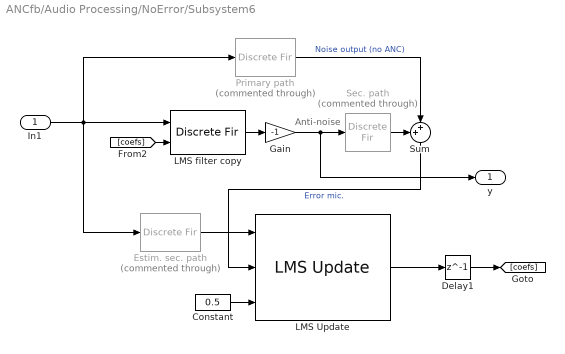
== system ANCfb/Audio Processing/NoError/Subsystem6 ==
  note: Anti-noise
  In1 : Inport
  Constant : Constant  Value=0.5
  Delay1 : Delay  DelayLength=1
  Estim. sec. path : DiscreteFir  Commented=through  Coefficients="[0.466  0.533  -0.257  -0.274  -0.231  -0.175]"
  Gain : Gain  Gain=-1
  LMS Update : dspadpt3/LMS Update  Method=Normalized LMS  Length=200  NumFilters=1  StepSizeSource=Input port  StepSize=0.1  LeakageFactor=1.0  InitialConditions=0  AdaptiveFilterMode=Tapped delay-line FIR filter  EnableAdaptInput=off  EnableResetInput=off  SimulateUsing=Interpreted execution
  LMS filter copy : DiscreteFir  CoefSource=Input port
      settings: InputPortMap=u0,u1
  Primary path : DiscreteFir  Commented=through  Coefficients=conv([0.5 0.5 -.3 -.3 -.2 -.2],[.1 -.1 .2 -.2 .3 -.3 .15 -.15])
  Sec. path : DiscreteFir  Commented=through  Coefficients=[0.5 0.5 -.3 -.3 -.2 -.2]
  Sum : Sum  Inputs=++|
  y : Outport
  wires:
  Primary path/1 -> Sum/2  "Noise output (no ANC)"
  Gain/1 -> y/1, Sec. path/1
  Constant/1 -> LMS Update/3
  LMS filter copy/1 -> Gain/1
  [coefs] -> LMS filter copy/2
  Sum/1 -> LMS Update/2  "Error mic."
  Delay1/1 -> [coefs]
  LMS Update/1 -> Delay1/1
  In1/1 -> Primary path/1, Estim. sec. path/1, LMS filter copy/1
  Estim. sec. path/1 -> LMS Update/1
  Sec. path/1 -> Sum/1

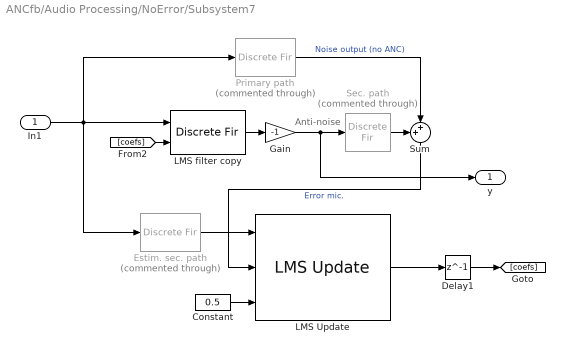
== system ANCfb/Audio Processing/NoError/Subsystem7 ==
  note: Anti-noise
  In1 : Inport
  Constant : Constant  Value=0.5
  Delay1 : Delay  DelayLength=1
  Estim. sec. path : DiscreteFir  Commented=through  Coefficients="[0.466  0.533  -0.257  -0.274  -0.231  -0.175]"
  Gain : Gain  Gain=-1
  LMS Update : dspadpt3/LMS Update  Method=Normalized LMS  Length=200  NumFilters=1  StepSizeSource=Input port  StepSize=0.1  LeakageFactor=1.0  InitialConditions=0  AdaptiveFilterMode=Tapped delay-line FIR filter  EnableAdaptInput=off  EnableResetInput=off  SimulateUsing=Interpreted execution
  LMS filter copy : DiscreteFir  CoefSource=Input port
      settings: InputPortMap=u0,u1
  Primary path : DiscreteFir  Commented=through  Coefficients=conv([0.5 0.5 -.3 -.3 -.2 -.2],[.1 -.1 .2 -.2 .3 -.3 .15 -.15])
  Sec. path : DiscreteFir  Commented=through  Coefficients=[0.5 0.5 -.3 -.3 -.2 -.2]
  Sum : Sum  Inputs=++|
  y : Outport
  wires:
  Primary path/1 -> Sum/2  "Noise output (no ANC)"
  Gain/1 -> y/1, Sec. path/1
  Constant/1 -> LMS Update/3
  LMS filter copy/1 -> Gain/1
  [coefs] -> LMS filter copy/2
  Sum/1 -> LMS Update/2  "Error mic."
  Delay1/1 -> [coefs]
  LMS Update/1 -> Delay1/1
  In1/1 -> Primary path/1, Estim. sec. path/1, LMS filter copy/1
  Estim. sec. path/1 -> LMS Update/1
  Sec. path/1 -> Sum/1

== system ANCfb/Audio Processing/NoError/Subsystem8 ==
  note: Anti-noise
  In1 : Inport
  Constant : Constant  Value=0.5
  Delay1 : Delay  DelayLength=1
  Estim. sec. path : DiscreteFir  Commented=through  Coefficients="[0.466  0.533  -0.257  -0.274  -0.231  -0.175]"
  Gain : Gain  Gain=-1
  LMS Update : dspadpt3/LMS Update  Method=Normalized LMS  Length=200  NumFilters=1  StepSizeSource=Input port  StepSize=0.1  LeakageFactor=1.0  InitialConditions=0  AdaptiveFilterMode=Tapped delay-line FIR filter  EnableAdaptInput=off  EnableResetInput=off  SimulateUsing=Interpreted execution
  LMS filter copy : DiscreteFir  CoefSource=Input port
      settings: InputPortMap=u0,u1
  Primary path : DiscreteFir  Commented=through  Coefficients=conv([0.5 0.5 -.3 -.3 -.2 -.2],[.1 -.1 .2 -.2 .3 -.3 .15 -.15])
  Sec. path : DiscreteFir  Commented=through  Coefficients=[0.5 0.5 -.3 -.3 -.2 -.2]
  Sum : Sum  Inputs=++|
  y : Outport
  wires:
  Primary path/1 -> Sum/2  "Noise output (no ANC)"
  Gain/1 -> y/1, Sec. path/1
  Constant/1 -> LMS Update/3
  LMS filter copy/1 -> Gain/1
  [coefs] -> LMS filter copy/2
  Sum/1 -> LMS Update/2  "Error mic."
  Delay1/1 -> [coefs]
  LMS Update/1 -> Delay1/1
  In1/1 -> Primary path/1, Estim. sec. path/1, LMS filter copy/1
  Estim. sec. path/1 -> LMS Update/1
  Sec. path/1 -> Sum/1

== system ANCfb/Audio Processing/NoError/Subsystem9 ==
  note: Anti-noise
  In1 : Inport
  Constant : Constant  Value=0.5
  Delay1 : Delay  DelayLength=1
  Estim. sec. path : DiscreteFir  Commented=through  Coefficients="[0.466  0.533  -0.257  -0.274  -0.231  -0.175]"
  Gain : Gain  Gain=-1
  LMS Update : dspadpt3/LMS Update  Method=Normalized LMS  Length=200  NumFilters=1  StepSizeSource=Input port  StepSize=0.1  LeakageFactor=1.0  InitialConditions=0  AdaptiveFilterMode=Tapped delay-line FIR filter  EnableAdaptInput=off  EnableResetInput=off  SimulateUsing=Interpreted execution
  LMS filter copy : DiscreteFir  CoefSource=Input port
      settings: InputPortMap=u0,u1
  Primary path : DiscreteFir  Commented=through  Coefficients=conv([0.5 0.5 -.3 -.3 -.2 -.2],[.1 -.1 .2 -.2 .3 -.3 .15 -.15])
  Sec. path : DiscreteFir  Commented=through  Coefficients=[0.5 0.5 -.3 -.3 -.2 -.2]
  Sum : Sum  Inputs=++|
  y : Outport
  wires:
  Primary path/1 -> Sum/2  "Noise output (no ANC)"
  Gain/1 -> y/1, Sec. path/1
  Constant/1 -> LMS Update/3
  LMS filter copy/1 -> Gain/1
  [coefs] -> LMS filter copy/2
  Sum/1 -> LMS Update/2  "Error mic."
  Delay1/1 -> [coefs]
  LMS Update/1 -> Delay1/1
  In1/1 -> Primary path/1, Estim. sec. path/1, LMS filter copy/1
  Estim. sec. path/1 -> LMS Update/1
  Sec. path/1 -> Sum/1

== system ANCfb/Audio Processing/Right Channel, exec/Subsystem ==
  note: Anti-noise
  In1 : Inport
  In2 : Inport  Port=2
  Constant : Constant  Value=0.5
  Delay1 : Delay  DelayLength=1
  Estim. sec. path : DiscreteFir  Commented=through  Coefficients="[0.466  0.533  -0.257  -0.274  -0.231  -0.175]"
  Gain : Gain  Gain=-1
  LMS Update : dspadpt3/LMS Update  Method=Normalized LMS  Length=L  NumFilters=1  StepSizeSource=Input port  StepSize=0.1  LeakageFactor=1.0  InitialConditions=0  AdaptiveFilterMode=Tapped delay-line FIR filter  EnableAdaptInput=off  EnableResetInput=off  SimulateUsing=Interpreted execution
  LMS filter copy : DiscreteFir  CoefSource=Input port
      settings: InputPortMap=u0,u1
  y : Outport
  wires:
  Gain/1 -> y/1
  Constant/1 -> LMS Update/3
  LMS filter copy/1 -> Gain/1
  [coefs] -> LMS filter copy/2
  Delay1/1 -> [coefs]
  LMS Update/1 -> Delay1/1
  In1/1 -> Estim. sec. path/1, LMS filter copy/1
  Estim. sec. path/1 -> LMS Update/1
  In2/1 -> LMS Update/2

== system ANCfb/Audio Processing/Right Channel, exec/Subsystem1 ==
  In1 : Inport
  In2 : Inport  Port=2
  Constant : Constant  Value=0.5
  Delay1 : Delay  DelayLength=1
  Estim. sec. path : DiscreteFir  Commented=through  Coefficients="[0.466  0.533  -0.257  -0.274  -0.231  -0.175]"
  Gain : Gain  Gain=-1
  LMS Update : dspadpt3/LMS Update  Method=Normalized LMS  Length=L  NumFilters=1  StepSizeSource=Input port  StepSize=0.1  LeakageFactor=1.0  InitialConditions=0  AdaptiveFilterMode=Tapped delay-line FIR filter  EnableAdaptInput=off  EnableResetInput=off  SimulateUsing=Interpreted execution
  LMS filter copy : DiscreteFir  CoefSource=Input port
      settings: InputPortMap=u0,u1
  y : Outport
  wires:
  Gain/1 -> y/1
  Constant/1 -> LMS Update/3
  LMS filter copy/1 -> Gain/1
  [coefs] -> LMS filter copy/2
  Delay1/1 -> [coefs]
  LMS Update/1 -> Delay1/1
  In1/1 -> Estim. sec. path/1, LMS filter copy/1
  Estim. sec. path/1 -> LMS Update/1
  In2/1 -> LMS Update/2

== system ANCfb/Audio Processing/Right Channel, exec/Subsystem2 ==
  In1 : Inport
  In2 : Inport  Port=2
  Constant : Constant  Value=0.5
  Delay1 : Delay  DelayLength=1
  Estim. sec. path : DiscreteFir  Commented=through  Coefficients="[0.466  0.533  -0.257  -0.274  -0.231  -0.175]"
  Gain : Gain  Gain=-1
  LMS Update : dspadpt3/LMS Update  Method=Normalized LMS  Length=L  NumFilters=1  StepSizeSource=Input port  StepSize=0.1  LeakageFactor=1.0  InitialConditions=0  AdaptiveFilterMode=Tapped delay-line FIR filter  EnableAdaptInput=off  EnableResetInput=off  SimulateUsing=Interpreted execution
  LMS filter copy : DiscreteFir  CoefSource=Input port
      settings: InputPortMap=u0,u1
  y : Outport
  wires:
  Gain/1 -> y/1
  Constant/1 -> LMS Update/3
  LMS filter copy/1 -> Gain/1
  [coefs] -> LMS filter copy/2
  Delay1/1 -> [coefs]
  LMS Update/1 -> Delay1/1
  In1/1 -> Estim. sec. path/1, LMS filter copy/1
  Estim. sec. path/1 -> LMS Update/1
  In2/1 -> LMS Update/2

== system ANCfb/Audio Processing/Right Channel, exec/Subsystem3 ==
  In1 : Inport
  In2 : Inport  Port=2
  Constant : Constant  Value=0.5
  Delay1 : Delay  DelayLength=1
  Estim. sec. path : DiscreteFir  Commented=through  Coefficients="[0.466  0.533  -0.257  -0.274  -0.231  -0.175]"
  Gain : Gain  Gain=-1
  LMS Update : dspadpt3/LMS Update  Method=Normalized LMS  Length=L  NumFilters=1  StepSizeSource=Input port  StepSize=0.1  LeakageFactor=1.0  InitialConditions=0  AdaptiveFilterMode=Tapped delay-line FIR filter  EnableAdaptInput=off  EnableResetInput=off  SimulateUsing=Interpreted execution
  LMS filter copy : DiscreteFir  CoefSource=Input port
      settings: InputPortMap=u0,u1
  y : Outport
  wires:
  Gain/1 -> y/1
  Constant/1 -> LMS Update/3
  LMS filter copy/1 -> Gain/1
  [coefs] -> LMS filter copy/2
  Delay1/1 -> [coefs]
  LMS Update/1 -> Delay1/1
  In1/1 -> Estim. sec. path/1, LMS filter copy/1
  Estim. sec. path/1 -> LMS Update/1
  In2/1 -> LMS Update/2

== system ANCfb/Audio Processing/Right Channel, exec/Subsystem4 ==
  In1 : Inport
  In2 : Inport  Port=2
  Constant : Constant  Value=0.5
  Delay1 : Delay  DelayLength=1
  Estim. sec. path : DiscreteFir  Commented=through  Coefficients="[0.466  0.533  -0.257  -0.274  -0.231  -0.175]"
  Gain : Gain  Gain=-1
  LMS Update : dspadpt3/LMS Update  Method=Normalized LMS  Length=L  NumFilters=1  StepSizeSource=Input port  StepSize=0.1  LeakageFactor=1.0  InitialConditions=0  AdaptiveFilterMode=Tapped delay-line FIR filter  EnableAdaptInput=off  EnableResetInput=off  SimulateUsing=Interpreted execution
  LMS filter copy : DiscreteFir  CoefSource=Input port
      settings: InputPortMap=u0,u1
  y : Outport
  wires:
  Gain/1 -> y/1
  Constant/1 -> LMS Update/3
  LMS filter copy/1 -> Gain/1
  [coefs] -> LMS filter copy/2
  Delay1/1 -> [coefs]
  LMS Update/1 -> Delay1/1
  In1/1 -> Estim. sec. path/1, LMS filter copy/1
  Estim. sec. path/1 -> LMS Update/1
  In2/1 -> LMS Update/2

== system ANCfb/Audio Processing/Right Channel, exec/Subsystem5 ==
  In1 : Inport
  In2 : Inport  Port=2
  Constant : Constant  Value=0.5
  Delay1 : Delay  DelayLength=1
  Estim. sec. path : DiscreteFir  Commented=through  Coefficients="[0.466  0.533  -0.257  -0.274  -0.231  -0.175]"
  Gain : Gain  Gain=-1
  LMS Update : dspadpt3/LMS Update  Method=Normalized LMS  Length=L  NumFilters=1  StepSizeSource=Input port  StepSize=0.1  LeakageFactor=1.0  InitialConditions=0  AdaptiveFilterMode=Tapped delay-line FIR filter  EnableAdaptInput=off  EnableResetInput=off  SimulateUsing=Interpreted execution
  LMS filter copy : DiscreteFir  CoefSource=Input port
      settings: InputPortMap=u0,u1
  y : Outport
  wires:
  Gain/1 -> y/1
  Constant/1 -> LMS Update/3
  LMS filter copy/1 -> Gain/1
  [coefs] -> LMS filter copy/2
  Delay1/1 -> [coefs]
  LMS Update/1 -> Delay1/1
  In1/1 -> Estim. sec. path/1, LMS filter copy/1
  Estim. sec. path/1 -> LMS Update/1
  In2/1 -> LMS Update/2

== system ANCfb/Audio Processing/Right Channel, exec/Subsystem6 ==
  In1 : Inport
  In2 : Inport  Port=2
  Constant : Constant  Value=0.5
  Delay1 : Delay  DelayLength=1
  Estim. sec. path : DiscreteFir  Commented=through  Coefficients="[0.466  0.533  -0.257  -0.274  -0.231  -0.175]"
  Gain : Gain  Gain=-1
  LMS Update : dspadpt3/LMS Update  Method=Normalized LMS  Length=L  NumFilters=1  StepSizeSource=Input port  StepSize=0.1  LeakageFactor=1.0  InitialConditions=0  AdaptiveFilterMode=Tapped delay-line FIR filter  EnableAdaptInput=off  EnableResetInput=off  SimulateUsing=Interpreted execution
  LMS filter copy : DiscreteFir  CoefSource=Input port
      settings: InputPortMap=u0,u1
  y : Outport
  wires:
  Gain/1 -> y/1
  Constant/1 -> LMS Update/3
  LMS filter copy/1 -> Gain/1
  [coefs] -> LMS filter copy/2
  Delay1/1 -> [coefs]
  LMS Update/1 -> Delay1/1
  In1/1 -> Estim. sec. path/1, LMS filter copy/1
  Estim. sec. path/1 -> LMS Update/1
  In2/1 -> LMS Update/2

== system ANCfb/Audio Processing/Right Channel, exec/Subsystem7 ==
  note: Anti-noise
  In1 : Inport
  In2 : Inport  Port=2
  Constant : Constant  Value=0.5
  Delay1 : Delay  DelayLength=1
  Estim. sec. path : DiscreteFir  Commented=through  Coefficients="[0.466  0.533  -0.257  -0.274  -0.231  -0.175]"
  Gain : Gain  Gain=-1
  LMS Update : dspadpt3/LMS Update  Method=Normalized LMS  Length=L  NumFilters=1  StepSizeSource=Input port  StepSize=0.1  LeakageFactor=1.0  InitialConditions=0  AdaptiveFilterMode=Tapped delay-line FIR filter  EnableAdaptInput=off  EnableResetInput=off  SimulateUsing=Interpreted execution
  LMS filter copy : DiscreteFir  CoefSource=Input port
      settings: InputPortMap=u0,u1
  y : Outport
  wires:
  Gain/1 -> y/1
  Constant/1 -> LMS Update/3
  LMS filter copy/1 -> Gain/1
  [coefs] -> LMS filter copy/2
  Delay1/1 -> [coefs]
  LMS Update/1 -> Delay1/1
  In1/1 -> Estim. sec. path/1, LMS filter copy/1
  Estim. sec. path/1 -> LMS Update/1
  In2/1 -> LMS Update/2

== system ANCfb/Audio Processing/Right Channel, exec/Subsystem8 ==
  note: Anti-noise
  In1 : Inport
  In2 : Inport  Port=2
  Constant : Constant  Value=0.5
  Delay1 : Delay  DelayLength=1
  Estim. sec. path : DiscreteFir  Commented=through  Coefficients="[0.466  0.533  -0.257  -0.274  -0.231  -0.175]"
  Gain : Gain  Gain=-1
  LMS Update : dspadpt3/LMS Update  Method=Normalized LMS  Length=L  NumFilters=1  StepSizeSource=Input port  StepSize=0.1  LeakageFactor=1.0  InitialConditions=0  AdaptiveFilterMode=Tapped delay-line FIR filter  EnableAdaptInput=off  EnableResetInput=off  SimulateUsing=Interpreted execution
  LMS filter copy : DiscreteFir  CoefSource=Input port
      settings: InputPortMap=u0,u1
  y : Outport
  wires:
  Gain/1 -> y/1
  Constant/1 -> LMS Update/3
  LMS filter copy/1 -> Gain/1
  [coefs] -> LMS filter copy/2
  Delay1/1 -> [coefs]
  LMS Update/1 -> Delay1/1
  In1/1 -> Estim. sec. path/1, LMS filter copy/1
  Estim. sec. path/1 -> LMS Update/1
  In2/1 -> LMS Update/2

== system ANCfb/Audio Processing/Right Channel, exec/Subsystem9 ==
  note: Anti-noise
  In1 : Inport
  In2 : Inport  Port=2
  Constant : Constant  Value=0.5
  Delay1 : Delay  DelayLength=1
  Estim. sec. path : DiscreteFir  Commented=through  Coefficients="[0.466  0.533  -0.257  -0.274  -0.231  -0.175]"
  Gain : Gain  Gain=-1
  LMS Update : dspadpt3/LMS Update  Method=Normalized LMS  Length=L  NumFilters=1  StepSizeSource=Input port  StepSize=0.1  LeakageFactor=1.0  InitialConditions=0  AdaptiveFilterMode=Tapped delay-line FIR filter  EnableAdaptInput=off  EnableResetInput=off  SimulateUsing=Interpreted execution
  LMS filter copy : DiscreteFir  CoefSource=Input port
      settings: InputPortMap=u0,u1
  y : Outport
  wires:
  Gain/1 -> y/1
  Constant/1 -> LMS Update/3
  LMS filter copy/1 -> Gain/1
  [coefs] -> LMS filter copy/2
  Delay1/1 -> [coefs]
  LMS Update/1 -> Delay1/1
  In1/1 -> Estim. sec. path/1, LMS filter copy/1
  Estim. sec. path/1 -> LMS Update/1
  In2/1 -> LMS Update/2

== system ANCfb/Audio Processing/Frame Breakdown/Subsystem/Subsystem ==
  note: Anti-noise
  In1 : Inport
  In2 : Inport  Port=2
  Delay : Delay  DelayLength=1  InitialCondition=0
  Delay1 : Delay  DelayLength=1
  Discrete FIR Filter : DiscreteFir  CoefSource=Input port
      settings: InputPortMap=u0,u1
  Estim. sec. path : DiscreteFir  Commented=through  Coefficients="[0.466  0.533  -0.257  -0.274  -0.231  -0.175]"
  Gain : Gain  Gain=-1
  LMS Update : dspadpt3/LMS Update  Method=Normalized LMS  Length=L  NumFilters=1  StepSizeSource=Property  StepSize=0.001  LeakageFactor=1.0  InitialConditions=0  AdaptiveFilterMode=Tapped delay-line FIR filter  EnableAdaptInput=off  EnableResetInput=off  SimulateUsing=Code generation
  LMS Update1 : dspadpt3/LMS Update  Method=LMS  Length=32  NumFilters=1  StepSizeSource=Property  StepSize=0.1  LeakageFactor=1.0  InitialConditions=0  AdaptiveFilterMode=Tapped delay-line FIR filter  EnableAdaptInput=off  EnableResetInput=off  SimulateUsing=Code generation
  LMS filter copy : DiscreteFir  CoefSource=Input port
      settings: InputPortMap=u0,u1
  Sum : Sum  Inputs=-+|
  y : Outport
  wires:
  Gain/1 -> LMS Update1/1, Delay/1, y/1
  LMS filter copy/1 -> Gain/1
  Delay1/1 -> LMS filter copy/2
  LMS Update/1 -> Delay1/1
  Estim. sec. path/1 -> LMS Update/1
  In2/1 -> LMS Update/2
  In1/1 -> Sum/2, LMS Update1/2
  LMS Update1/1 -> Discrete FIR Filter/2
  Delay/1 -> Discrete FIR Filter/1
  Discrete FIR Filter/1 -> Sum/1
  Sum/1 -> Estim. sec. path/1, LMS filter copy/1
